simulink model "cruise_control"  (R2016b)
settings: Solver=VariableStepAuto  StartTime=0.0  StopTime=10.0  RelTol=1e-3
PreLoadFcn:
  | load('cruise_control.mat');
values from neighbouring files (symbols this model uses):
  Ki = 1    [cruise_control.mat]
  Kp = 1    [cruise_control.mat]
settings Model: Creator=bartb  LastModifiedBy=bartb

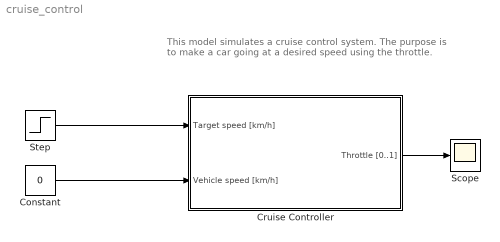
== system cruise_control ==
  note: This model simulates a cruise control system.
      | The purpose is to make a car going at a desired
      | speed using the throttle.
  Constant : Constant  Value=0
  Cruise Controller : Subsystem
  Scope : Scope
  Step : Step  After=0.1  SampleTime=0
  wires:
  Step/1 -> Cruise Controller/1(Target speed [km/h])
  Constant/1 -> Cruise Controller/2(Vehicle speed [km/h])
  Cruise Controller/1(Throttle [0..1]) -> Scope/1

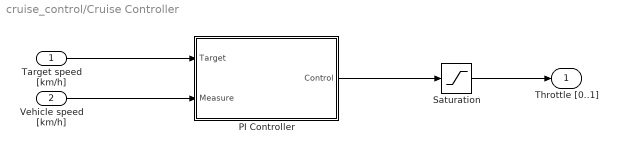
== system cruise_control/Cruise Controller ==
  Target speed [km/h] : Inport
  Vehicle speed [km/h] : Inport  Port=2
  PI Controller : Subsystem
  Saturation : Saturate
  Throttle [0..1] : Outport
  wires:
  Saturation/1 -> Throttle [0..1]/1
  Vehicle speed [km/h]/1 -> PI Controller/2(Measure)
  Target speed [km/h]/1 -> PI Controller/1(Target)
  PI Controller/1(Control) -> Saturation/1

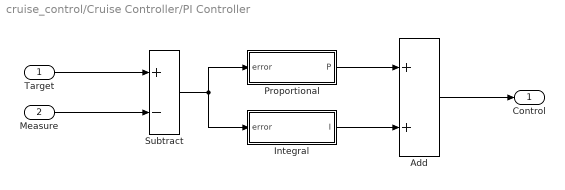
== system cruise_control/Cruise Controller/PI Controller ==
  Target : Inport
  Measure : Inport  Port=2
  Add : Sum
  Integral : Subsystem
  Proportional : Subsystem
  Subtract : Sum  Inputs=+-
  Control : Outport
  wires:
  Subtract/1 -> Integral/1(error), Proportional/1(error)
  Integral/1(I) -> Add/2
  Measure/1 -> Subtract/2
  Add/1 -> Control/1
  Target/1 -> Subtract/1
  Proportional/1(P) -> Add/1

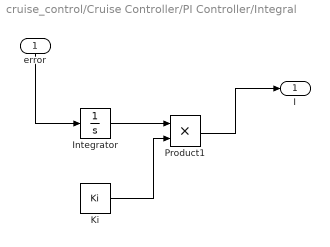
== system cruise_control/Cruise Controller/PI Controller/Integral ==
  error : Inport
  Integrator : Integrator
  Ki : Constant  Value=Ki
  Product1 : Product
  I : Outport
  wires:
  Product1/1 -> I/1
  Integrator/1 -> Product1/1
  Ki/1 -> Product1/2
  error/1 -> Integrator/1

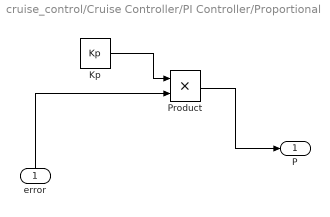
== system cruise_control/Cruise Controller/PI Controller/Proportional ==
  error : Inport
  Kp : Constant  Value=Kp
  Product : Product
  P : Outport
  wires:
  Kp/1 -> Product/1
  Product/1 -> P/1
  error/1 -> Product/2
